simulink model "SST_JOY_TITHI"  (R2019a)
settings: Solver=VariableStepAuto  StartTime=0.0  StopTime=10  RelTol=1e-3
libraries: powerlib x76, simulink x1
settings Model: Creator=JOY  LastModifiedBy=JOY

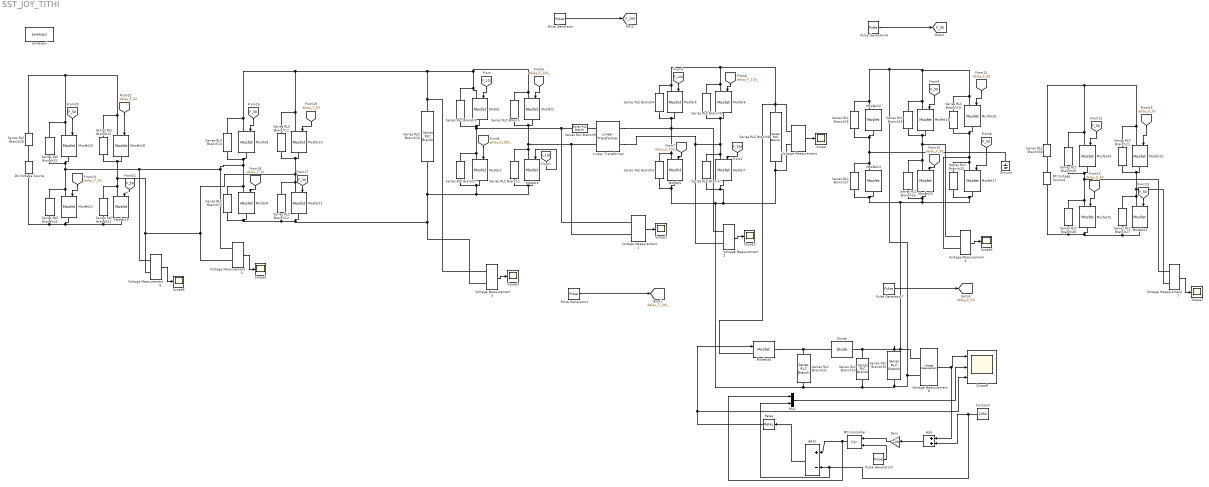
== system SST_JOY_TITHI ==
  Add : Sum
  Add1 : Sum  Inputs=+-
  Constant : Constant  Value=1050
  DC Voltage Source : powerlib/Electrical Sources/DC Voltage Source  Amplitude=1000  Measurements=None
      settings: SourceProductName=Simscape Electrical
  DC Voltage Source1 : powerlib/Electrical Sources/DC Voltage Source  Amplitude=1000  Measurements=None
      settings: SourceProductName=Simscape Electrical
  Diode : powerlib/Power Electronics/Diode  Ron=0.001  Lon=0  Vf=0.8  IC=0  UseSnubber=off  Rs=500  Cs=250e-9  Measurements=off
      settings: SourceProductName=Simscape Electrical
  Gain : Gain  Gain=100
  Ground : powerlib/Elements/Ground  LConnTagsString=a
      settings: SourceProductName=Simscape Electrical
  Linear Transformer : powerlib/Elements/Linear Transformer  UNITS=pu  NominalPower=[ 250e6 1000000 ]  winding1="[ 100e3  0.02  0.08 ]"  winding2="[ 100e3  0.02  0.08 ]"  ThreeWindings=off  winding3="[ 315e3  0.002  0.08 ]"  RmLm=[ 500e6 500e6 ]  Measurements=None  DataType=off
      settings: SourceProductName=Simscape Electrical
  Mosfet{,1..26} (27 alike) : powerlib/Power Electronics/Mosfet  Ron=0.1  Lon=0  Rd=0.01  Vfd=0  IC=0  Rs=1e5  Cs=inf  Measurements=off
      settings: SourceProductName=Simscape Electrical
  Mux : Mux  Inputs=2
  PID Controller : simulink/Continuous/PID Controller  Controller=I  Form=Parallel  TimeDomain=Continuous-time  SampleTime=-1  IntegratorMethod=Forward Euler  FilterMethod=Forward Euler  ControllerParametersSource=internal  P=1  I=40000  D=0  UseFilter=on  N=100  TunerSelectOption=Transfer Function Based (PID Tuner App)  InitialConditionSource=internal  InitialConditionForIntegrator=0  InitialConditionForFilter=0  DifferentiatorICPrevScaledInput=0  ExternalReset=rising  TrackingMode=off  Kt=1  LimitOutput=off  UpperSaturationLimit=inf  LowerSaturationLimit=-inf  LinearizeAsGain=on  AntiWindupMode=none  Kb=1  POutMin=[]  POutMax=[]  IOutMin=[]  IOutMax=[]  DOutMin=[]  DOutMax=[]  NOutMin=[]  NOutMax=[]  SumOutMin=[]  SumOutMax=[]  SaturationOutMin=[]  SaturationOutMax=[]  PParamMin=[]  PParamMax=[]  IParamMin=[]  IParamMax=[]  DParamMin=[]  DParamMax=[]  NParamMin=[]  NParamMax=[]  KbParamMin=[]  KbParamMax=[]  KtParamMin=[]  KtParamMax=[]  KbOutMin=[]  KbOutMax=[]  KtOutMin=[]  KtOutMax=[]  IntegratorOutMin=[]  IntegratorOutMax=[]  FilterOutMin=[]  FilterOutMax=[]  SumI1OutMin=[]  SumI1OutMax=[]  SumI2OutMin=[]  SumI2OutMax=[]  SumI3OutMin=[]  SumI3OutMax=[]  SumI4OutMin=[]  SumI4OutMax=[]  SumDOutMin=[]  SumDOutMax=[]  DifferentiatorOutMin=[]  DifferentiatorOutMax=[]  FilterDiffOutCoefMin=[]  FilterDiffOutCoefMax=[]  ReciprocalOutMin=[]  ReciprocalOutMax=[]  SumDenOutMin=[]  SumDenOutMax=[]  SumNumOutMin=[]  SumNumOutMax=[]  DivideOutMin=[]  DivideOutMax=[]  IntegratorContinuousStateAttributes=''  IntegratorStateMustResolveToSignalObject=off  IntegratorRTWStateStorageClass=Auto  FilterContinuousStateAttributes=''  FilterStateMustResolveToSignalObject=off  FilterRTWStateStorageClass=Auto  ParallelPVariant=Disabled  IdealPVariant=Disabled  IVariant=InternalParameters  DVariant=Disabled  IntegratorVariant=Continuous  SatVariant=Disabled  AWVariant=Passthrough  PCopyVariant=Disabled  TRVariant=Disabled  FdbkBlocksVariant=Forward  IdealPFdbkVariant=Disabled  SatFdbkVariant=Disabled  DerivativeFilterVariant=Disabled  NVariant=Disabled  NCopyVariant=Disabled_SignalSpec  FilterICVariant=Disabled  IntegratorICVariant=InternalICs  ExternalResetVariant=ExternalReset  TRSumVariant=Passthrough  SumFdbkVariant=Disabled  SumVariant=Passthrough_I
  Pulse Generator : DiscretePulseGenerator  PulseType=Time based  Period=1e-4  PulseWidth=50
  Pulse Generator1 : DiscretePulseGenerator  PulseType=Time based  Period=1e-4  PulseWidth=50  PhaseDelay=0.5e-4
  Pulse Generator2 : DiscretePulseGenerator  PulseType=Time based  Period=1/10000  PulseWidth=50
  Pulse Generator6 : DiscretePulseGenerator  PulseType=Time based  Period=2e-2  PulseWidth=50
  Pulse Generator7 : DiscretePulseGenerator  PulseType=Time based  Period=2e-2  PulseWidth=50  PhaseDelay=1e-2
  Relay : Relay
  Scope{,1..7} (8 alike) : Scope
  Scope8 : Scope  NumInputPorts=3
  Series RLC Branch{,1..7,11..25,27..29} (26 alike) : powerlib/Elements/Series RLC Branch  LConnTagsString=__new0  RConnTagsString=__new0  BranchType=C  Resistance=1  Inductance=1e-3  SetiL0=off  InitialCurrent=0  Capacitance=1e-6  Setx0=off  InitialVoltage=0  Measurements=None
      settings: SourceProductName=Simscape Electrical
  Series RLC Branch10 : powerlib/Elements/Series RLC Branch  LConnTagsString=__new0  RConnTagsString=__new0  BranchType=C  Resistance=1  Inductance=1e-3  SetiL0=off  InitialCurrent=0  Capacitance=1e-3  Setx0=off  InitialVoltage=0  Measurements=None
      settings: SourceProductName=Simscape Electrical
  Series RLC Branch26 : powerlib/Elements/Series RLC Branch  LConnTagsString=__new0  RConnTagsString=__new0  BranchType=R  Resistance=1  Inductance=1e-3  SetiL0=off  InitialCurrent=0  Capacitance=1e-6  Setx0=off  InitialVoltage=0  Measurements=None
      settings: SourceProductName=Simscape Electrical
  Series RLC Branch30 : powerlib/Elements/Series RLC Branch  LConnTagsString=__new0  RConnTagsString=__new0  BranchType=R  Resistance=1  Inductance=1e-3  SetiL0=off  InitialCurrent=0  Capacitance=1e-6  Setx0=off  InitialVoltage=0  Measurements=None
      settings: SourceProductName=Simscape Electrical
  Series RLC Branch31 : powerlib/Elements/Series RLC Branch  LConnTagsString=__new0  RConnTagsString=__new0  BranchType=L  Resistance=1  Inductance=10e-6  SetiL0=off  InitialCurrent=0  Capacitance=1e-6  Setx0=off  InitialVoltage=0  Measurements=None
      settings: SourceProductName=Simscape Electrical
  Series RLC Branch32 : powerlib/Elements/Series RLC Branch  LConnTagsString=__new0  RConnTagsString=__new0  BranchType=R  Resistance=100  Inductance=1e-3  SetiL0=off  InitialCurrent=0  Capacitance=1e-6  Setx0=off  InitialVoltage=0  Measurements=None
      settings: SourceProductName=Simscape Electrical
  Series RLC Branch33 : powerlib/Elements/Series RLC Branch  LConnTagsString=__new0  RConnTagsString=__new0  BranchType=C  Resistance=1  Inductance=1e-3  SetiL0=off  InitialCurrent=0  Capacitance=40e-3  Setx0=off  InitialVoltage=0  Measurements=None
      settings: SourceProductName=Simscape Electrical
  Series RLC Branch8 : powerlib/Elements/Series RLC Branch  LConnTagsString=__new0  RConnTagsString=__new0  BranchType=C  Resistance=1  Inductance=1e-3  SetiL0=off  InitialCurrent=0  Capacitance=1e-3  Setx0=off  InitialVoltage=0  Measurements=None
      settings: SourceProductName=Simscape Electrical
  Series RLC Branch9 : powerlib/Elements/Series RLC Branch  LConnTagsString=__new0  RConnTagsString=__new0  BranchType=L  Resistance=1  Inductance=200e-6  SetiL0=off  InitialCurrent=0  Capacitance=1e-6  Setx0=off  InitialVoltage=0  Measurements=None
      settings: SourceProductName=Simscape Electrical
  Voltage Measurement{,1..8} (9 alike) : powerlib/Measurements/Voltage Measurement  PhasorSimulation=off  OutputType=Complex  PSBequivalent=0
      settings: SourceProductName=Simscape Electrical
  powergui : powerlib/powergui  Priority=1  SimulationMode=Discrete  SampleTime=1.5e-5  frequency=60  Iterations=50  frequencyindice=0  Pbase=100e6  ErrMax=1e-4  UnitsV=kV  UnitsW=MW  buscounter=0  FunctionMessages=off  echomessages=off  EnableUseOfTLC=off  CurrentSourceSwitches=off  DisableSnubberDevices=off  DisableRonSwitches=off  DisableVfSwitches=off  DisplayEquations=off  AutomaticDiscreteSolvers=off  SolverType=Tustin/Backward Euler (TBE)  Interpol=off  ExternalGateDelay=off  methode=off  Ts=100  x0status=blocks  SPID=on  SwTol=0  HookPort=off  NonlinearTolerance=0  nMaxIteration=15  ContinueOnMaxIteration=off  RestoreLinks=warning  ResistiveCurrentMeasurement=off  Frange=[0:2:500]  Ylog=off  Xlog=on  ShowGrid=off  save=off  variable=ZData  structure=0  ZoomFFT=off  StartTime=0.0  cycles=1  DisplayStyle=1  fundamental=60  FreqAxis=off  MaxFrequency=1000  frequencyindicesteady=1  RmsSteady=1  display=off
      settings: SourceProductName=Simscape Electrical
  tag scope: F_100=global, F_50=global, delay_F_100_=global, delay_F_50=global
  wires:
  Voltage Measurement2/1 -> Scope2/1
  Voltage Measurement/1 -> Scope/1
  Pulse Generator/1 -> [F_100]
  Voltage Measurement1/1 -> Scope1/1
  Voltage Measurement3/1 -> Scope3/1
  Pulse Generator1/1 -> [delay_F_100_]
  Voltage Measurement4/1 -> Scope4/1
  Voltage Measurement5/1 -> Scope5/1
  Voltage Measurement6/1 -> Scope6/1
  Pulse Generator6/1 -> [F_50]
  Pulse Generator7/1 -> [delay_F_50]
  Voltage Measurement7/1 -> Scope7/1
  [F_100] -> Mosfet/1
  [F_100] -> Mosfet3/1
  [F_100] -> Mosfet7/1
  [F_100] -> Mosfet4/1
  [delay_F_100_] -> Mosfet1/1
  [delay_F_100_] -> Mosfet2/1
  [delay_F_100_] -> Mosfet6/1
  [delay_F_100_] -> Mosfet5/1
  [F_50] -> Mosfet17/1
  [F_50] -> Mosfet14/1
  [delay_F_50] -> Mosfet15/1
  [delay_F_50] -> Mosfet16/1
  [F_50] -> Mosfet24/1
  [F_50] -> Mosfet23/1
  [delay_F_50] -> Mosfet25/1
  [delay_F_50] -> Mosfet22/1
  [F_50] -> Mosfet8/1
  [F_50] -> Mosfet11/1
  [delay_F_50] -> Mosfet9/1
  [delay_F_50] -> Mosfet10/1
  [F_50] -> Mosfet20/1
  [F_50] -> Mosfet19/1
  [delay_F_50] -> Mosfet18/1
  [delay_F_50] -> Mosfet21/1
  Relay/1 -> Mosfet26/1, Scope8/3
  Mux/1 -> Scope8/2
  Pulse Generator2/1 -> PID Controller/2
  Add1/1 -> Relay/1
  PID Controller/1 -> Add1/1, Mux/1
  Constant/1 -> Mux/2, Add1/2, Add/2
  Gain/1 -> PID Controller/1
  Voltage Measurement8/1 -> Add/1, Scope8/1
  Add/1 -> Gain/1
  connections:
  Linear Transformer/RConn2 -- Voltage Measurement2/LConn2 -- Mosfet6/RConn1 -- Series RLC Branch6/LConn1 -- Series RLC Branch7/RConn1 -- Mosfet7/LConn1
  Series RLC Branch9/LConn1 -- Voltage Measurement1/LConn1 -- Mosfet/RConn1 -- Series RLC Branch3/LConn1 -- Series RLC Branch2/RConn1 -- Mosfet1/LConn1
  Mosfet2/LConn1 -- Voltage Measurement3/LConn1 -- Series RLC Branch10/RConn1 -- Series RLC Branch14/RConn1 -- Mosfet8/LConn1 -- Series RLC Branch11/RConn1 -- Mosfet10/LConn1 -- Series RLC Branch3/RConn1 -- Mosfet/LConn1 -- Series RLC Branch/RConn1
  Series RLC Branch2/LConn1 -- Series RLC Branch10/LConn1 -- Voltage Measurement3/LConn2 -- Series RLC Branch13/LConn1 -- Mosfet9/RConn1 -- Series RLC Branch12/LConn1 -- Mosfet11/RConn1 -- Series RLC Branch1/LConn1 -- Mosfet3/RConn1 -- Mosfet1/RConn1
  Linear Transformer/RConn1 -- Mosfet4/RConn1 -- Series RLC Branch4/LConn1 -- Voltage Measurement2/LConn1 -- Series RLC Branch5/RConn1 -- Mosfet5/LConn1
  Mosfet3/LConn1 -- Mosfet2/RConn1 -- Series RLC Branch/LConn1 -- Voltage Measurement1/LConn2 -- Linear Transformer/LConn2 -- Series RLC Branch1/RConn1
  Series RLC Branch9/RConn1 -- Linear Transformer/LConn1
  Voltage Measurement7/LConn2 -- Mosfet22/RConn1 -- Series RLC Branch21/LConn1 -- Series RLC Branch27/RConn1 -- Mosfet23/LConn1
  Series RLC Branch18/LConn1 -- Mosfet12/RConn1 -- Series RLC Branch17/RConn1 -- Mosfet13/LConn1 -- Ground/LConn1
  Series RLC Branch13/RConn1 -- Mosfet9/LConn1 -- Voltage Measurement5/LConn1 -- Series RLC Branch24/RConn1 -- Mosfet21/LConn1 -- Mosfet20/RConn1 -- Series RLC Branch25/LConn1 -- Voltage Measurement6/LConn1 -- Mosfet8/RConn1 -- Series RLC Branch14/LConn1
  Mosfet21/RConn1 -- DC Voltage Source/LConn1 -- Series RLC Branch24/LConn1 -- Series RLC Branch23/LConn1 -- Mosfet19/RConn1
  Mosfet18/LConn1 -- Series RLC Branch22/RConn1 -- Series RLC Branch26/LConn1 -- Series RLC Branch25/RConn1 -- Mosfet20/LConn1
  DC Voltage Source/RConn1 -- Series RLC Branch26/RConn1
  Series RLC Branch28/LConn1 -- DC Voltage Source1/LConn1 -- Mosfet25/RConn1 -- Series RLC Branch27/LConn1 -- Mosfet23/RConn1
  Mosfet24/LConn1 -- Mosfet22/LConn1 -- Series RLC Branch21/RConn1 -- Series RLC Branch30/LConn1 -- Series RLC Branch29/RConn1
  DC Voltage Source1/RConn1 -- Series RLC Branch30/RConn1
  Mosfet11/LConn1 -- Mosfet18/RConn1 -- Series RLC Branch22/LConn1 -- Series RLC Branch23/RConn1 -- Mosfet19/LConn1 -- Voltage Measurement6/LConn2 -- Voltage Measurement5/LConn2 -- Mosfet10/RConn1 -- Series RLC Branch11/LConn1 -- Series RLC Branch12/RConn1
  Series RLC Branch29/LConn1 -- Mosfet24/RConn1 -- Voltage Measurement7/LConn1 -- Series RLC Branch28/RConn1 -- Mosfet25/LConn1
  Series RLC Branch15/LConn1 -- Mosfet14/RConn1 -- Voltage Measurement4/LConn1 -- Series RLC Branch16/RConn1 -- Mosfet15/LConn1
  Mosfet16/RConn1 -- Voltage Measurement4/LConn2 -- Mosfet17/LConn1 -- Series RLC Branch20/RConn1 -- Series RLC Branch19/LConn1
  Series RLC Branch31/LConn1 -- Mosfet26/RConn1 -- Diode/RConn1
  Series RLC Branch8/RConn1 -- Mosfet26/LConn1 -- Mosfet6/LConn1 -- Series RLC Branch6/RConn1 -- Series RLC Branch4/RConn1 -- Mosfet4/LConn1 -- Voltage Measurement/LConn1
  Series RLC Branch32/LConn1 -- Series RLC Branch20/LConn1 -- Mosfet17/RConn1 -- Series RLC Branch16/LConn1 -- Mosfet15/RConn1 -- Series RLC Branch17/LConn1 -- Mosfet13/RConn1 -- Voltage Measurement8/LConn1 -- Diode/LConn1 -- Series RLC Branch33/LConn1
  Mosfet5/RConn1 -- Mosfet7/RConn1 -- Series RLC Branch7/LConn1 -- Series RLC Branch8/LConn1 -- Voltage Measurement/LConn2 -- Series RLC Branch31/RConn1 -- Series RLC Branch18/RConn1 -- Mosfet12/LConn1 -- Series RLC Branch19/RConn1 -- Mosfet16/LConn1 -- Series RLC Branch15/RConn1 -- Mosfet14/LConn1 -- Voltage Measurement8/LConn2 -- Series RLC Branch32/RConn1 -- Series RLC Branch33/RConn1 -- Series RLC Branch5/LConn1
